simulink model "heat_pump"  (R2024a)
settings: Solver=VariableStepAuto  StartTime=0.0  StopTime=3600*24*2  RelTol=1e-3
settings Model: Creator=ml4  LastModifiedBy=ml4

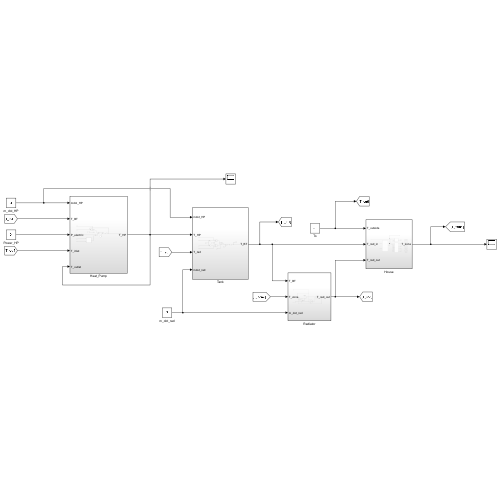
[thumbnail: Simulink's stored preview of the top-level diagram]
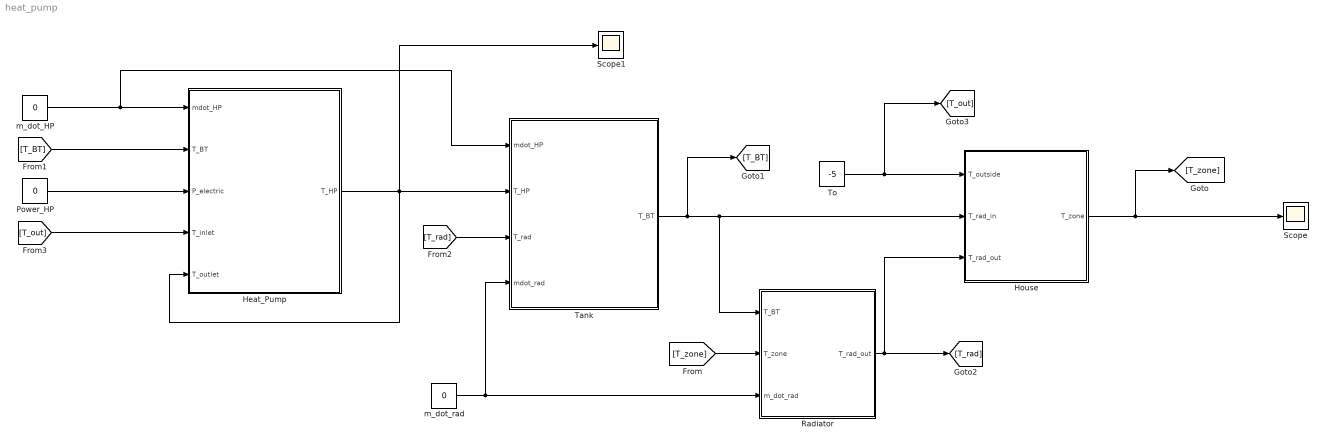
== system heat_pump ==
  Heat_Pump : Subsystem
  House : Subsystem
  Power_HP : Constant  Value=0
  Radiator : Subsystem
  Scope : Scope
  Scope1 : Scope
  Tank : Subsystem
  To : Constant  Value=-5
  m_dot_HP : Constant  Value=0
  m_dot_rad : Constant  Value=0
  wires:
  To/1 -> [T_out], House/1(T_outside)
  House/1(T_zone) -> Scope/1, [T_zone]
  [T_zone] -> Radiator/2(T_zone)
  m_dot_rad/1 -> Tank/4(mdot_rad), Radiator/3(m_dot_rad)
  Radiator/1(T_rad_out) -> [T_rad], House/3(T_rad_out)
  Tank/1(T_BT) -> [T_BT], Radiator/1(T_BT), House/2(T_rad_in)
  m_dot_HP/1 -> Tank/1(mdot_HP), Heat_Pump/1(mdot_HP)
  [T_rad] -> Tank/3(T_rad)
  [T_BT] -> Heat_Pump/2(T_BT)
  Power_HP/1 -> Heat_Pump/3(P_electric)
  [T_out] -> Heat_Pump/4(T_inlet)
  Heat_Pump/1(T_HP) -> Heat_Pump/5(T_outlet), Scope1/1, Tank/2(T_HP)

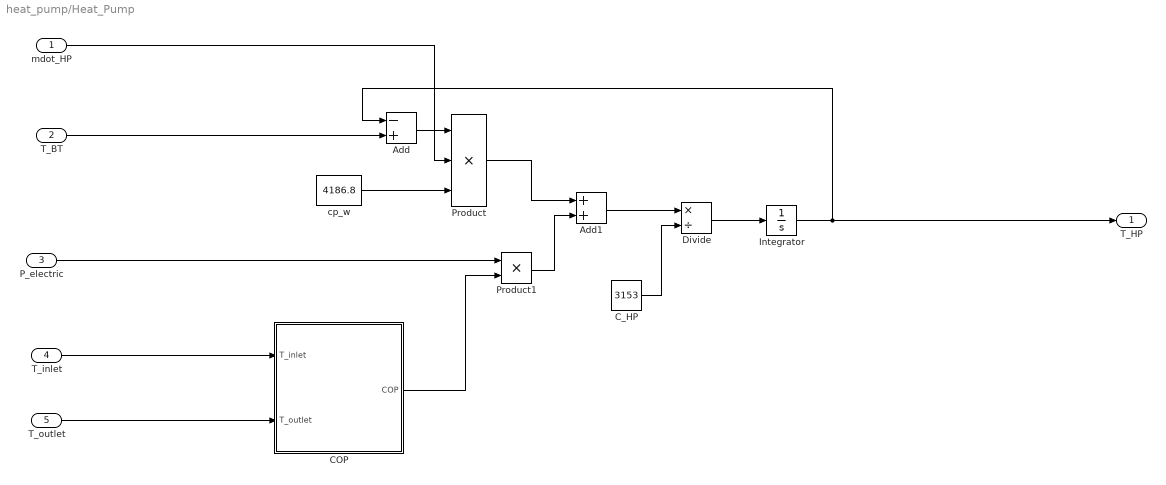
== system heat_pump/Heat_Pump ==
  mdot_HP : Inport
  T_BT : Inport  Port=2
  P_electric : Inport  Port=3
  T_inlet : Inport  Port=4
  T_outlet : Inport  Port=5
  Add : Sum  Inputs=-+
  Add1 : Sum
  COP : Subsystem
  C_HP : Constant  Value=3153
  Divide : Product  Inputs=*/
  Integrator : Integrator  InitialCondition=60
  Product : Product  Inputs=3
  Product1 : Product
  cp_w : Constant  Value=4186.8
  T_HP : Outport
  wires:
  Product1/1 -> Add1/2
  C_HP/1 -> Divide/2
  Add/1 -> Product/1
  Product/1 -> Add1/1
  Divide/1 -> Integrator/1
  Integrator/1 -> T_HP/1, Add/1
  cp_w/1 -> Product/3
  Add1/1 -> Divide/1
  mdot_HP/1 -> Product/2
  T_BT/1 -> Add/2
  COP/1(COP) -> Product1/2
  T_inlet/1 -> COP/1(T_inlet)
  P_electric/1 -> Product1/1
  T_outlet/1 -> COP/2(T_outlet)

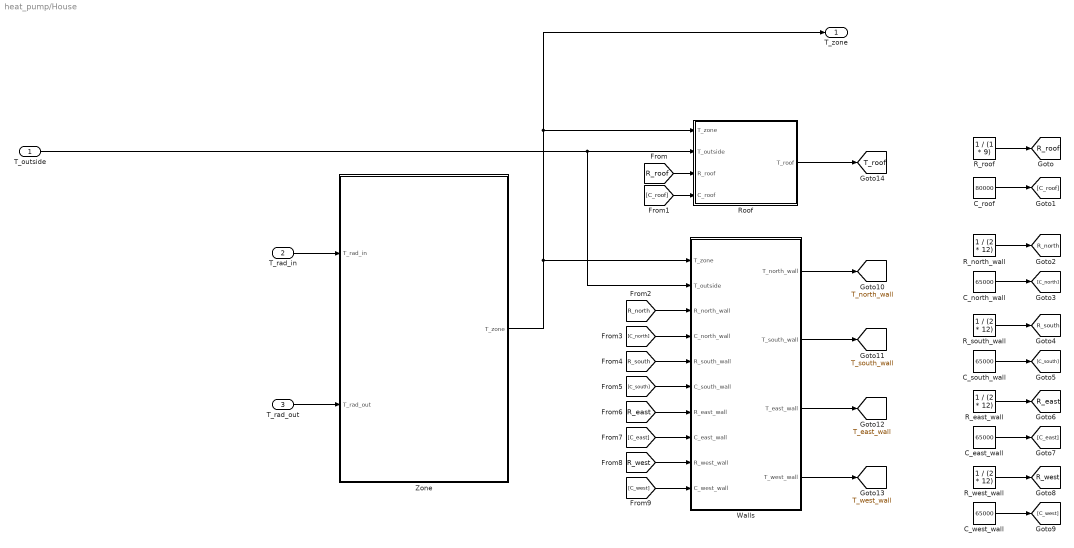
== system heat_pump/House ==
  T_outside : Inport
  T_rad_in : Inport  Port=2
  T_rad_out : Inport  Port=3
  C_east_wall : Constant  Value=65000
  C_north_wall : Constant  Value=65000
  C_roof : Constant  Value=80000
  C_south_wall : Constant  Value=65000
  C_west_wall : Constant  Value=65000
  R_east_wall : Constant  Value=1 / (2 * 12)
  R_north_wall : Constant  Value=1 / (2 * 12)
  R_roof : Constant  Value=1 / (1 * 9)
  R_south_wall : Constant  Value=1 / (2 * 12)
  R_west_wall : Constant  Value=1 / (2 * 12)
  Roof : Subsystem
  Walls : Subsystem
  Zone : Subsystem
  T_zone : Outport
  tag scope: R_east=global, R_north=global, R_roof=global, R_south=global, R_west=global, T_east_wall=global, T_north_wall=global, T_roof=global, T_south_wall=global, T_west_wall=global
  wires:
  [R_west] -> Walls/9(R_west_wall)
  Walls/3(T_east_wall) -> [T_east_wall]
  [R_east] -> Walls/7(R_east_wall)
  C_roof/1 -> [C_roof]
  C_east_wall/1 -> [C_east]
  [C_west] -> Walls/10(C_west_wall)
  C_south_wall/1 -> [C_south]
  R_north_wall/1 -> [R_north]
  Walls/1(T_north_wall) -> [T_north_wall]
  T_outside/1 -> Walls/2(T_outside), Roof/2(T_outside)
  [R_south] -> Walls/5(R_south_wall)
  C_west_wall/1 -> [C_west]
  T_rad_in/1 -> Zone/1(T_rad_in)
  [C_north] -> Walls/4(C_north_wall)
  Roof/1(T_roof) -> [T_roof]
  [C_east] -> Walls/8(C_east_wall)
  [R_north] -> Walls/3(R_north_wall)
  R_east_wall/1 -> [R_east]
  R_roof/1 -> [R_roof]
  Walls/4(T_west_wall) -> [T_west_wall]
  [C_roof] -> Roof/4(C_roof)
  R_west_wall/1 -> [R_west]
  R_south_wall/1 -> [R_south]
  Walls/2(T_south_wall) -> [T_south_wall]
  [R_roof] -> Roof/3(R_roof)
  Zone/1(T_zone) -> T_zone/1, Roof/1(T_zone), Walls/1(T_zone)
  C_north_wall/1 -> [C_north]
  [C_south] -> Walls/6(C_south_wall)
  T_rad_out/1 -> Zone/2(T_rad_out)

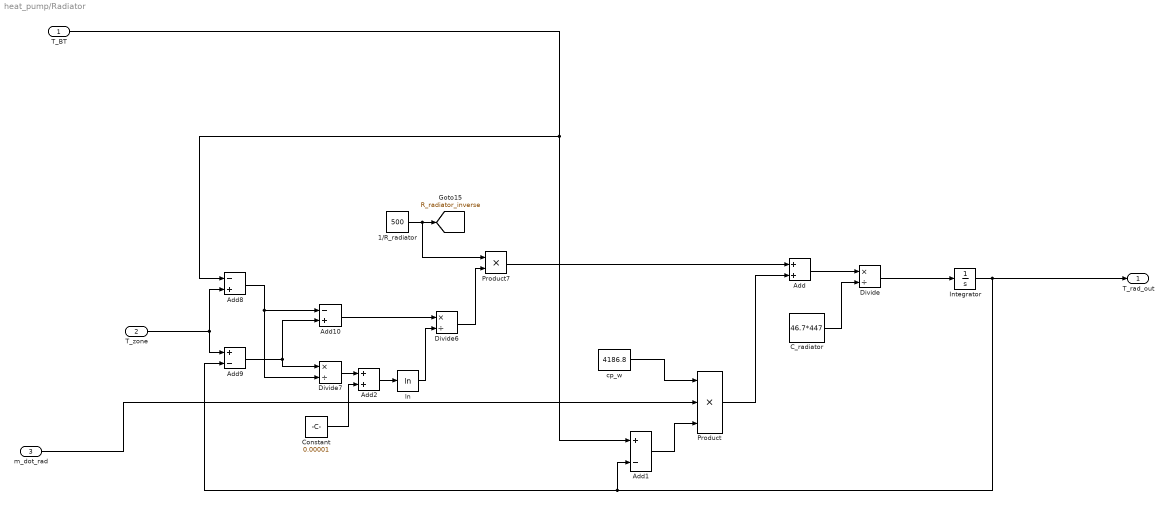
== system heat_pump/Radiator ==
  T_BT : Inport
  T_zone : Inport  Port=2
  m_dot_rad : Inport  Port=3
  1/R_radiator : Constant  Value=500
  Add : Sum
  Add1 : Sum  Inputs=+-
  Add10 : Sum  Inputs=-+
  Add2 : Sum
  Add8 : Sum  Inputs=-+
  Add9 : Sum  Inputs=+-
  C_radiator : Constant  Value=46.7*447
  Constant : Constant  Value=0.00001
  Divide : Product  Inputs=*/
  Divide6 : Product  Inputs=*/
  Divide7 : Product  Inputs=*/
  Integrator : Integrator  InitialCondition=20
  Product : Product  Inputs=3
  Product7 : Product
  cp_w : Constant  Value=4186.8
  ln : Math  Operator=log
  T_rad_out : Outport
  tag scope: R_radiator_inverse=global
  wires:
  1/R_radiator/1 -> Product7/1, [R_radiator_inverse]
  T_zone/1 -> Add9/1, Add8/2
  Integrator/1 -> T_rad_out/1, Add1/2, Add9/2
  Product7/1 -> Add/1
  T_BT/1 -> Add1/1, Add8/1
  Add1/1 -> Product/3
  Divide6/1 -> Product7/2
  Add8/1 -> Divide7/2, Add10/1
  C_radiator/1 -> Divide/2
  Add9/1 -> Divide7/1, Add10/2
  Divide/1 -> Integrator/1
  Product/1 -> Add/2
  cp_w/1 -> Product/1
  ln/1 -> Divide6/2
  Add10/1 -> Divide6/1
  Add/1 -> Divide/1
  m_dot_rad/1 -> Product/2
  Divide7/1 -> Add2/1
  Add2/1 -> ln/1
  Constant/1 -> Add2/2

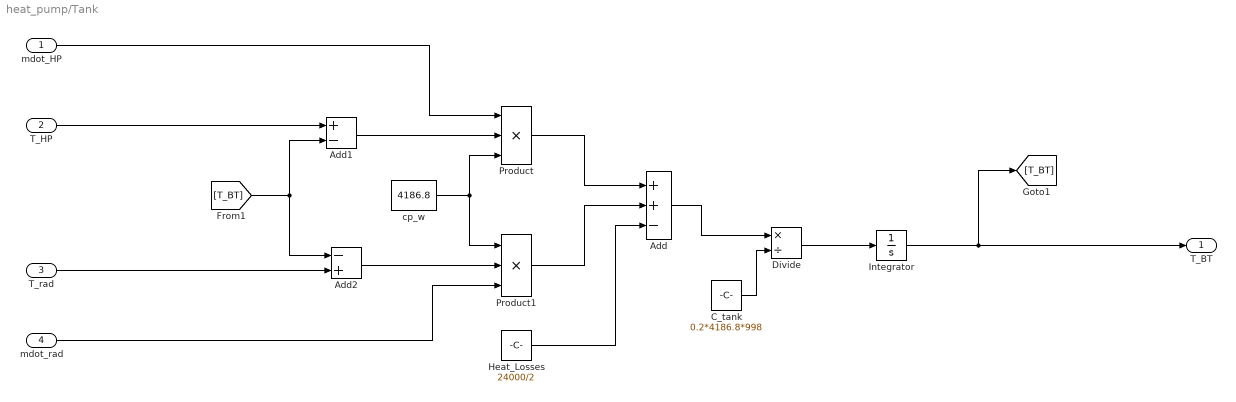
== system heat_pump/Tank ==
  mdot_HP : Inport
  T_HP : Inport  Port=2
  T_rad : Inport  Port=3
  mdot_rad : Inport  Port=4
  Add : Sum  Inputs=++-
  Add1 : Sum  Inputs=+-
  Add2 : Sum  Inputs=-+
  C_tank : Constant  Value=0.2*4186.8*998
  Divide : Product  Inputs=*/
  Heat_Losses : Constant  Value=24000/2
  Integrator : Integrator  InitialCondition=50
  Product : Product  Inputs=3
  Product1 : Product  Inputs=3
  cp_w : Constant  Value=4186.8
  T_BT : Outport
  wires:
  mdot_rad/1 -> Product1/3
  [T_BT] -> Add2/1, Add1/2
  mdot_HP/1 -> Product/1
  Product1/1 -> Add/2
  Divide/1 -> Integrator/1
  Integrator/1 -> T_BT/1, [T_BT]
  Add1/1 -> Product/2
  cp_w/1 -> Product1/1, Product/3
  Add/1 -> Divide/1
  Add2/1 -> Product1/2
  Product/1 -> Add/1
  C_tank/1 -> Divide/2
  T_HP/1 -> Add1/1
  Heat_Losses/1 -> Add/3
  T_rad/1 -> Add2/2

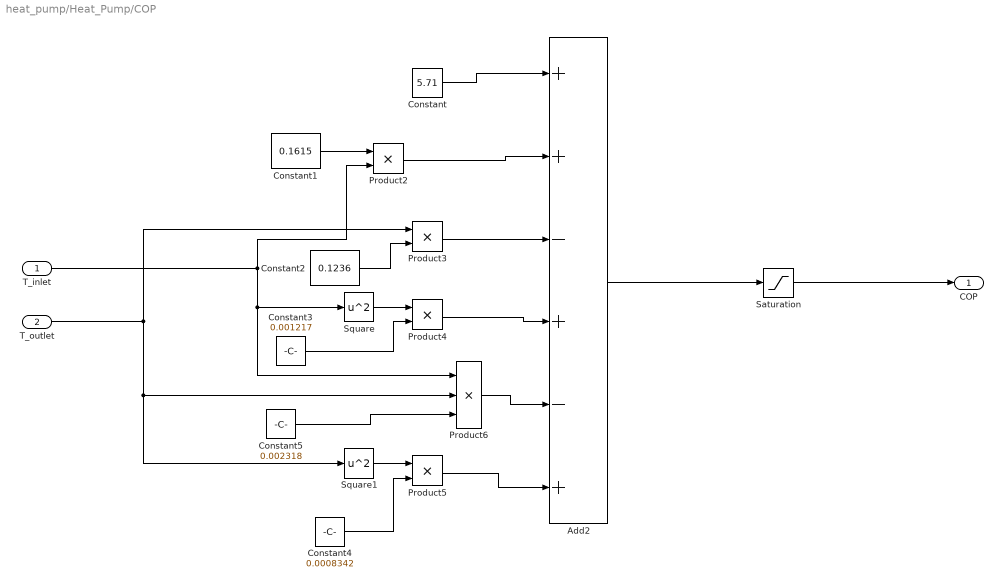
== system heat_pump/Heat_Pump/COP ==
  T_inlet : Inport
  T_outlet : Inport  Port=2
  Add2 : Sum  Inputs=++-+-+
  Constant : Constant  Value=5.71
  Constant1 : Constant  Value=0.1615
  Constant2 : Constant  Value=0.1236
  Constant3 : Constant  Value=0.001217
  Constant4 : Constant  Value=0.0008342
  Constant5 : Constant  Value=0.002318
  Product{2..5} (4 alike) : Product
  Product6 : Product  Inputs=3
  Saturation : Saturate  UpperLimit=4.9  LowerLimit=1.1
  Square : Math  Operator=square
  Square1 : Math  Operator=square
  COP : Outport
  wires:
  Constant5/1 -> Product6/3
  Product3/1 -> Add2/3
  T_outlet/1 -> Product3/1, Product6/2, Square1/1
  T_inlet/1 -> Product2/2, Product6/1, Square/1
  Product2/1 -> Add2/2
  Product4/1 -> Add2/4
  Product5/1 -> Add2/6
  Constant3/1 -> Product4/2
  Square/1 -> Product4/1
  Constant1/1 -> Product2/1
  Constant2/1 -> Product3/2
  Constant/1 -> Add2/1
  Constant4/1 -> Product5/2
  Square1/1 -> Product5/1
  Product6/1 -> Add2/5
  Add2/1 -> Saturation/1
  Saturation/1 -> COP/1

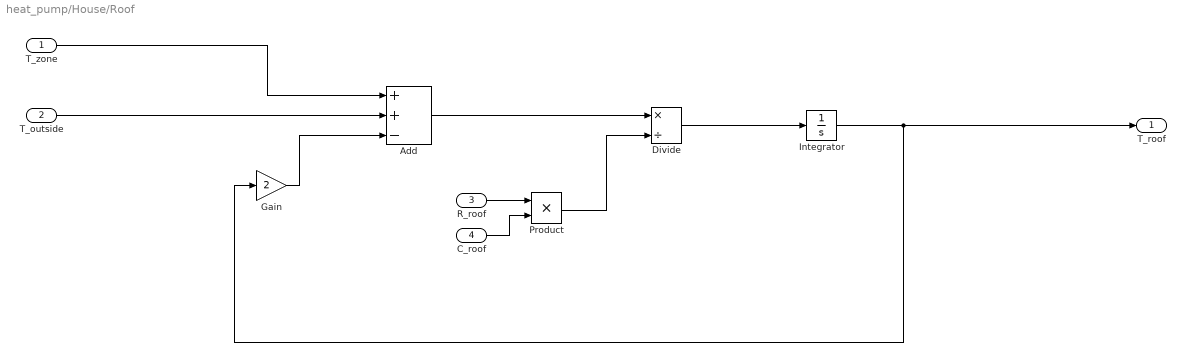
== system heat_pump/House/Roof ==
  T_zone : Inport
  T_outside : Inport  Port=2
  R_roof : Inport  Port=3
  C_roof : Inport  Port=4
  Add : Sum  Inputs=++-
  Divide : Product  Inputs=*/
  Gain : Gain  Gain=2
  Integrator : Integrator
  Product : Product
  T_roof : Outport
  wires:
  T_zone/1 -> Add/1
  Integrator/1 -> T_roof/1, Gain/1
  Product/1 -> Divide/2
  Gain/1 -> Add/3
  Divide/1 -> Integrator/1
  Add/1 -> Divide/1
  T_outside/1 -> Add/2
  R_roof/1 -> Product/1
  C_roof/1 -> Product/2

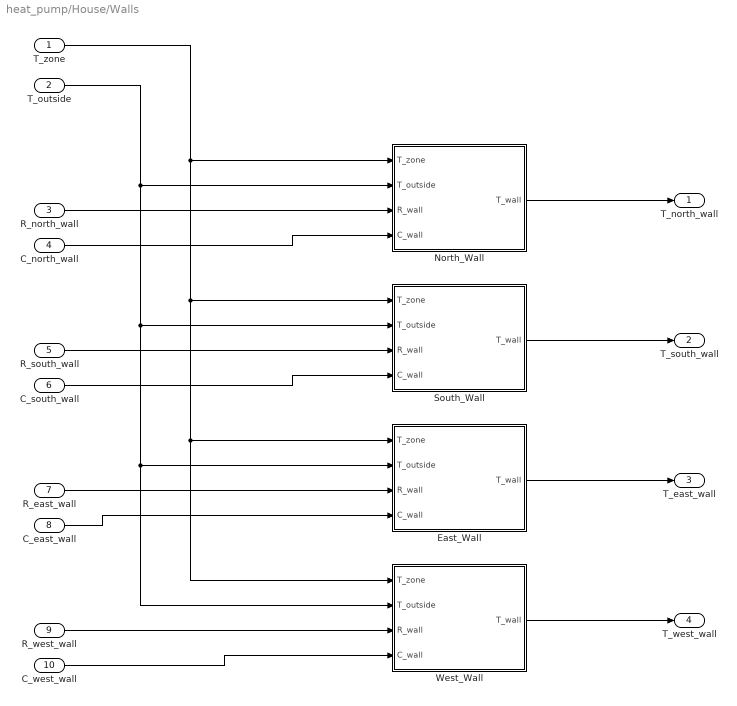
== system heat_pump/House/Walls ==
  T_zone : Inport
  T_outside : Inport  Port=2
  R_north_wall : Inport  Port=3
  C_north_wall : Inport  Port=4
  R_south_wall : Inport  Port=5
  C_south_wall : Inport  Port=6
  R_east_wall : Inport  Port=7
  C_east_wall : Inport  Port=8
  R_west_wall : Inport  Port=9
  C_west_wall : Inport  Port=10
  East_Wall : Subsystem
  North_Wall : Subsystem
  South_Wall : Subsystem
  West_Wall : Subsystem
  T_north_wall : Outport
  T_south_wall : Outport  Port=2
  T_east_wall : Outport  Port=3
  T_west_wall : Outport  Port=4
  wires:
  T_outside/1 -> North_Wall/2(T_outside), South_Wall/2(T_outside), East_Wall/2(T_outside), West_Wall/2(T_outside)
  T_zone/1 -> North_Wall/1(T_zone), South_Wall/1(T_zone), East_Wall/1(T_zone), West_Wall/1(T_zone)
  West_Wall/1(T_wall) -> T_west_wall/1
  South_Wall/1(T_wall) -> T_south_wall/1
  East_Wall/1(T_wall) -> T_east_wall/1
  North_Wall/1(T_wall) -> T_north_wall/1
  R_north_wall/1 -> North_Wall/3(R_wall)
  C_north_wall/1 -> North_Wall/4(C_wall)
  R_south_wall/1 -> South_Wall/3(R_wall)
  C_south_wall/1 -> South_Wall/4(C_wall)
  R_east_wall/1 -> East_Wall/3(R_wall)
  C_east_wall/1 -> East_Wall/4(C_wall)
  R_west_wall/1 -> West_Wall/3(R_wall)
  C_west_wall/1 -> West_Wall/4(C_wall)

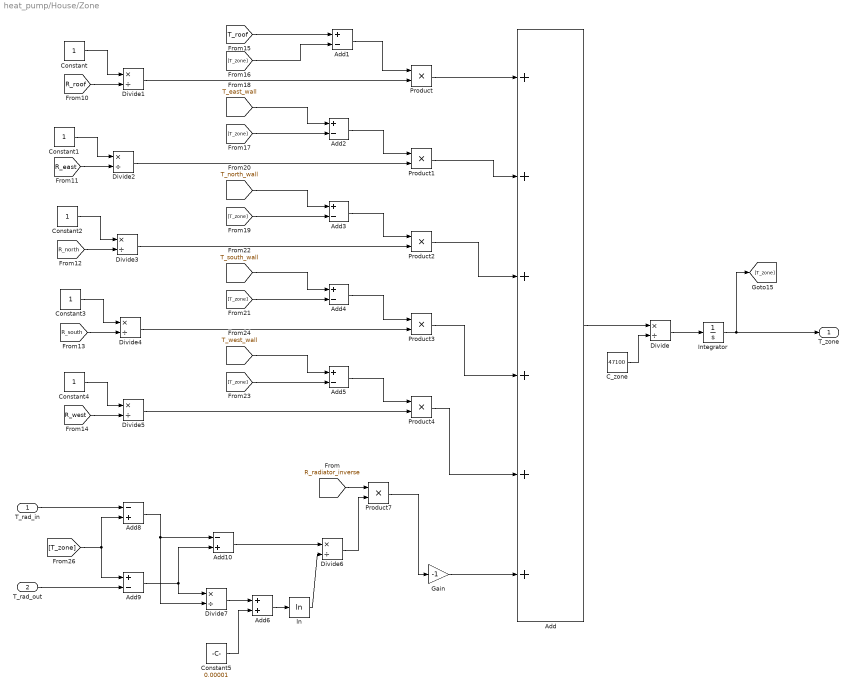
== system heat_pump/House/Zone ==
  T_rad_in : Inport
  T_rad_out : Inport  Port=2
  Add : Sum  Inputs=++++++
  Add{1..5,9} (6 alike) : Sum  Inputs=+-
  Add10 : Sum  Inputs=-+
  Add6 : Sum
  Add8 : Sum  Inputs=-+
  C_zone : Constant  Value=47100
  Constant{,1..4} (5 alike) : Constant
  Constant5 : Constant  Value=0.00001
  Divide{,1..7} (8 alike) : Product  Inputs=*/
  Gain : Gain  Gain=-1
  Integrator : Integrator  InitialCondition=10
  Product{,1..4,7} (6 alike) : Product
  ln : Math  Operator=log
  T_zone : Outport
  wires:
  Product2/1 -> Add/3
  Divide3/1 -> Product2/2
  Add/1 -> Divide/1
  [R_roof] -> Divide1/2
  T_rad_in/1 -> Add8/1
  C_zone/1 -> Divide/2
  [T_east_wall] -> Add2/1
  Add9/1 -> Divide7/1, Add10/2
  Constant3/1 -> Divide4/1
  [T_zone] -> Add2/2
  Integrator/1 -> T_zone/1, [T_zone]
  T_rad_out/1 -> Add9/2
  [R_east] -> Divide2/2
  Product7/1 -> Gain/1
  Constant2/1 -> Divide3/1
  Constant1/1 -> Divide2/1
  Constant/1 -> Divide1/1
  Product1/1 -> Add/2
  [T_south_wall] -> Add4/1
  [R_south] -> Divide4/2
  [T_zone] -> Add1/2
  Product3/1 -> Add/4
  Divide2/1 -> Product1/2
  Add4/1 -> Product3/1
  Divide/1 -> Integrator/1
  Product/1 -> Add/1
  [T_west_wall] -> Add5/1
  [T_north_wall] -> Add3/1
  [R_north] -> Divide3/2
  Add1/1 -> Product/1
  [T_roof] -> Add1/1
  Divide6/1 -> Product7/2
  Divide1/1 -> Product/2
  Add10/1 -> Divide6/1
  [T_zone] -> Add3/2
  Constant4/1 -> Divide5/1
  [T_zone] -> Add4/2
  Add8/1 -> Divide7/2, Add10/1
  Add2/1 -> Product1/1
  [T_zone] -> Add9/1, Add8/2
  [T_zone] -> Add5/2
  Divide5/1 -> Product4/2
  Add3/1 -> Product2/1
  Add5/1 -> Product4/1
  Divide4/1 -> Product3/2
  [R_west] -> Divide5/2
  Product4/1 -> Add/5
  ln/1 -> Divide6/2
  [R_radiator_inverse] -> Product7/1
  Gain/1 -> Add/6
  Constant5/1 -> Add6/2
  Divide7/1 -> Add6/1
  Add6/1 -> ln/1

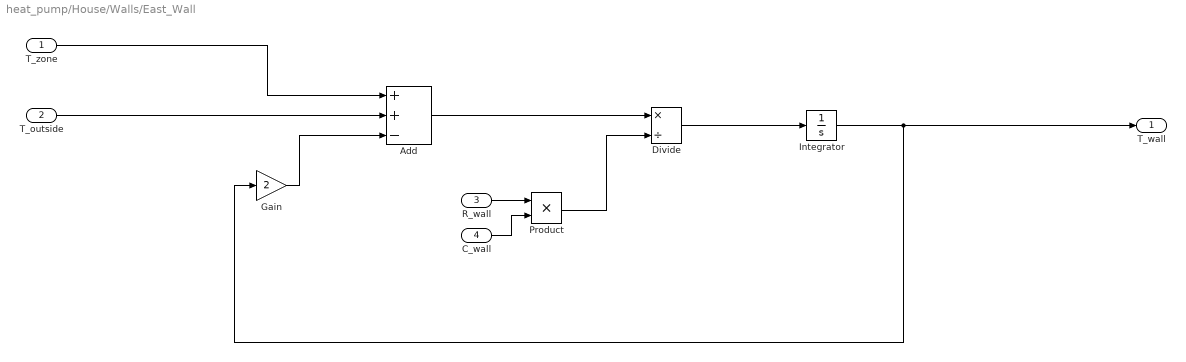
== system heat_pump/House/Walls/East_Wall ==
  T_zone : Inport
  T_outside : Inport  Port=2
  R_wall : Inport  Port=3
  C_wall : Inport  Port=4
  Add : Sum  Inputs=++-
  Divide : Product  Inputs=*/
  Gain : Gain  Gain=2
  Integrator : Integrator
  Product : Product
  T_wall : Outport
  wires:
  T_outside/1 -> Add/2
  Add/1 -> Divide/1
  Divide/1 -> Integrator/1
  Gain/1 -> Add/3
  Product/1 -> Divide/2
  Integrator/1 -> Gain/1, T_wall/1
  T_zone/1 -> Add/1
  R_wall/1 -> Product/1
  C_wall/1 -> Product/2

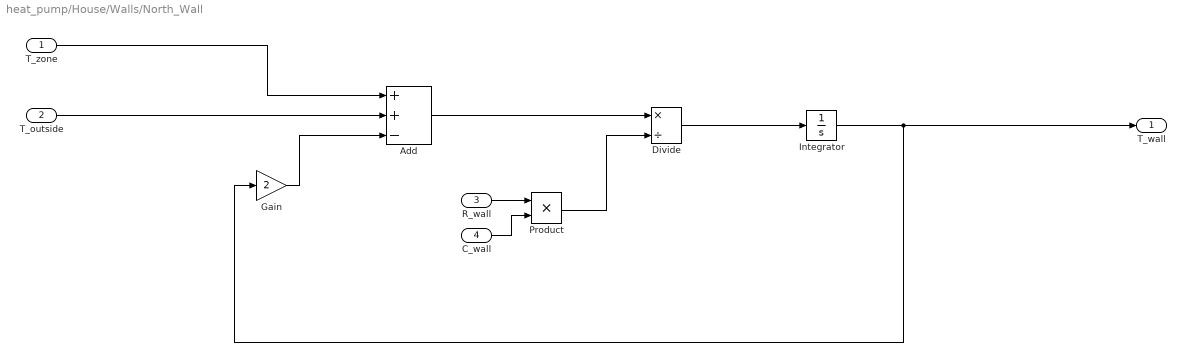
== system heat_pump/House/Walls/North_Wall ==
  T_zone : Inport
  T_outside : Inport  Port=2
  R_wall : Inport  Port=3
  C_wall : Inport  Port=4
  Add : Sum  Inputs=++-
  Divide : Product  Inputs=*/
  Gain : Gain  Gain=2
  Integrator : Integrator
  Product : Product
  T_wall : Outport
  wires:
  T_outside/1 -> Add/2
  Add/1 -> Divide/1
  Divide/1 -> Integrator/1
  Gain/1 -> Add/3
  Product/1 -> Divide/2
  Integrator/1 -> Gain/1, T_wall/1
  T_zone/1 -> Add/1
  R_wall/1 -> Product/1
  C_wall/1 -> Product/2

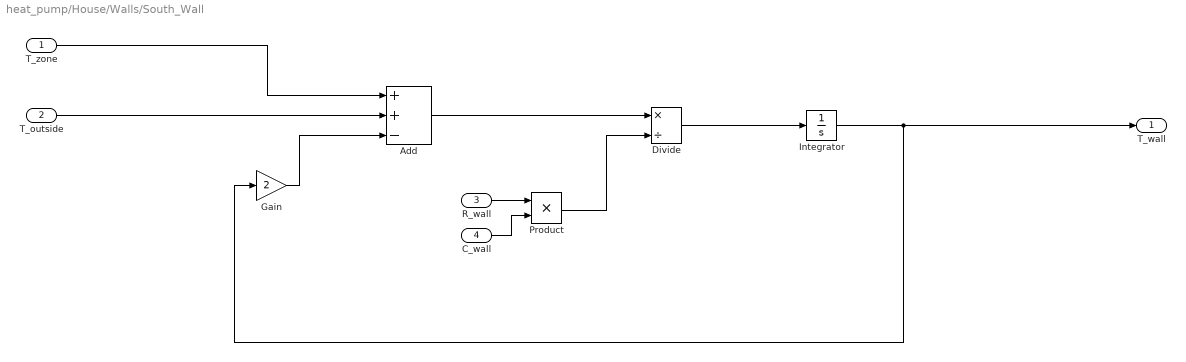
== system heat_pump/House/Walls/South_Wall ==
  T_zone : Inport
  T_outside : Inport  Port=2
  R_wall : Inport  Port=3
  C_wall : Inport  Port=4
  Add : Sum  Inputs=++-
  Divide : Product  Inputs=*/
  Gain : Gain  Gain=2
  Integrator : Integrator
  Product : Product
  T_wall : Outport
  wires:
  C_wall/1 -> Product/2
  R_wall/1 -> Product/1
  T_zone/1 -> Add/1
  Integrator/1 -> T_wall/1, Gain/1
  Product/1 -> Divide/2
  Gain/1 -> Add/3
  Divide/1 -> Integrator/1
  Add/1 -> Divide/1
  T_outside/1 -> Add/2

== system heat_pump/House/Walls/West_Wall ==
  T_zone : Inport
  T_outside : Inport  Port=2
  R_wall : Inport  Port=3
  C_wall : Inport  Port=4
  Add : Sum  Inputs=++-
  Divide : Product  Inputs=*/
  Gain : Gain  Gain=2
  Integrator : Integrator
  Product : Product
  T_wall : Outport
  wires:
  C_wall/1 -> Product/2
  R_wall/1 -> Product/1
  T_zone/1 -> Add/1
  Integrator/1 -> T_wall/1, Gain/1
  Product/1 -> Divide/2
  Gain/1 -> Add/3
  Divide/1 -> Integrator/1
  Add/1 -> Divide/1
  T_outside/1 -> Add/2
